simulink model "nmm2DFullBody"  (R2018a)
settings: Solver=ode23s  StartTime=0.0  StopTime=13  FixedStep=1e-3  MaxStep=ts_max  RelTol=1e-3  AbsTol=1e-4  EnableMultiTasking=on
InitFcn:
  | addpath('../lib');
  | addpath('./init_script');
  | nms_model_MechInit
  | nms_model_ControlInit
StopFcn:
  | mRFX = struct;
  | 
  | mRFX.RStance = DataFromModel.Data(:,2)
  | mRFX.RGRF_AP = DataFromModel.Data(:,24)
  | mRFX.RGRF_VT = DataFromModel.Data(:,22)
  | mRFX.RAnkleAngle = DataFromModel.Data(:,8)
  | mRFX.RKneeAngle = DataFromModel.Data(:,7)
  | mRFX.RHipAngle = DataFromModel.Data(:,6)
  | mRFX.RAnkleTorque = DataFromModel.Data(:,20)
  | mRFX.RKneeTorque = DataFromModel.Data(:,19)
  | mRFX.RHipTorque = DataFromModel.Data(:,18)
  | 
  | mRFX.RMuscleGLU = DataFromModel.Data(:,32)
  | mRFX.RMuscleHF = DataFromModel.Data(:,33)
  | mRFX.RMuscleHAM = DataFromModel.Data(:,34)
  | mRFX.RMuscleVAS = DataFromModel.Data(:,35)
  | mRFX.RMuscleGAS = DataFromModel.Data(:,36)
  | mRFX.RMuscleSOL = DataFromModel.Data(:,37)
  | mRFX.RMuscleTA = DataFromModel.Data(:,38)
  | 
  | mRFX.LStance = DataFromModel.Data(:,1)
  | mRFX.LGRF_AP = DataFromModel.Data(:,23)
  | mRFX.LGRF_VT = DataFromModel.Data(:,21)
  | mRFX.LAnkleAngle = DataFromModel.Data(:,5)
  | mRFX.LKneeAngle = DataFromModel.Data(:,4)
  | mRFX.LHipAngle = DataFromModel.Data(:,3)
  | mRFX.LAnkleTorque = DataFromModel.Data(:,17)
  | mRFX.LKneeTorque = DataFromModel.Data(:,16)
  | mRFX.LHipTorque = DataFromModel.Data(:,15)
  | 
  | mRFX.LMuscleGLU = DataFromModel.Data(:,25)
  | mRFX.LMuscleHF = DataFromModel.Data(:,26)
  | mRFX.LMuscleHAM = DataFromModel.Data(:,27)
  | mRFX.LMuscleVAS = DataFromModel.Data(:,28)
  | mRFX.LMuscleGAS = DataFromModel.Data(:,29)
  | mRFX.LMuscleSOL = DataFromModel.Data(:,30)
  | mRFX.LMuscleTA = DataFromModel.Data(:,31)
undefined symbols (not defined in the file or in its folder): alphaFmGas, alphaFmGlu, alphaFmHam, alphaFmSol, alphaFmVas, alphaLceHam, alphaLceHfl, alphaLceTa, alphaLceTa1, Amp, amp_var, c, c_jointstop, D12_F, D12_S, D12_T, D13_F, D1G_F, D1G_HAT, D1G_S, D1G_T, DeltaThRef, eref, FmaxGAS, FmaxGLU, FmaxHAM, FmaxHFL, FmaxSOL, FmaxTA, FmaxVAS, freq, freq_var, GainDeltaTheta, GainGAS, GainGLU, GainHAM, GainHAMHFL, GainHFL, GainKneOverExt, GainSOL, GainSOLTA, GainTA, GainVAS, In_F, In_HAT, In_S, In_T, K, k_gx, k_gy, k_pressure, K_swing, LceOffsetHAM, LceOffsetHFL, LceOffsetTA, LongDelay, loptGAS, loptGLU, loptHAM, loptHFL ... (+83)
libraries: nmc x77, mblibv1 x60, simulink x33, simulink_extras x18
(part 1 of 8)
settings Model: SimulationMode=accelerator  Creator=hgeyer  LastModifiedBy=Alice
settings SolverCC: AutoScaleAbsTol=off
settings DataIOCC: LimitDataPoints=on  MaxDataPoints=2500  SaveFormat=Array  SignalLoggingSaveFormat=ModelDataLogs  SaveState=on  SignalLogging=off  StateSaveName=xoutNew  OutputSaveName=youtNew
settings OptimizationCC: BooleanDataType=off  ExpressionDepthLimit=2147483647  InitFltsAndDblsToZero=on  EfficientMapNaN2IntZero=off  LifeSpan=inf
settings DebuggingCC: SaveWithParameterizedLinksMsg=none  UnderspecifiedInitializationDetection=Classic  MergeDetectMultiDrivingBlocksExec=none  SignalResolutionControl=TryResolveAllWithWarning  SolverPrmCheckMsg=warning  MultiTaskDSMMsg=warning  MultiTaskCondExecSysMsg=none  FcnCallInpInsideContextMsg=warning  AllowSymbolicDim=off  StateNameClashWarn=warning  SFUnexpectedBacktrackingDiag=warning  SFNoUnconditionalDefaultTransitionDiag=warning  SFExecutionAtInitializationDiag=none
settings HardwareCC: ProdBitPerPointer=32  ProdBitPerSizeT=32  ProdBitPerPtrDiffT=32  ProdLargestAtomicFloat=None  ProdIntDivRoundTo=Undefined  ProdEndianess=Unspecified  ProdWordSize=32  ProdHWDeviceType=32-bit Generic  TargetBitPerPointer=64  TargetBitPerSizeT=64  TargetBitPerPtrDiffT=64  TargetLongLongMode=on  TargetIntDivRoundTo=Zero  TargetEndianess=LittleEndian  TargetWordSize=64  TargetHWDeviceType=MATLAB Host  ProdEqTarget=off
settings ModelReferenceCC: PropagateSignalLabelsOutOfModel=off
settings CodeAppCC: MaxIdLength=128  StateflowObjectComments=on
settings GRTTargetCC: TargetLangStandard=C89/C90 (ANSI)  CombineOutputUpdateFcns=off  GRTInterface=on
settings ConfigComp: CovMetricSettings=dw  CovHtmlReporting=on  CovSaveCumulativeToWorkspaceVar=on  CovSaveSingleToWorkspaceVar=on  CovExternalEMLEnable=off  CovSFcnEnable=off
settings SimMechanicsCC: VisDuringSimulation=on  VisSampleTime=0.01  AutoFitVis=TIGHTFIT  LastVizWinPosition=[551 264 570 413]  CamPosition=[16.8615;0.833613;11.9413;]  CamTarget=[16.8615;0.833613;0;]  CamUpVector=[0;1;0;]  CamHeight=1.70989  VisBackgroundColor=[0.9;0.9;0.95;]  DefaultBodyColor=[1;0;0;]
settings ConfigurationSet: Description=SimMechanics 2G

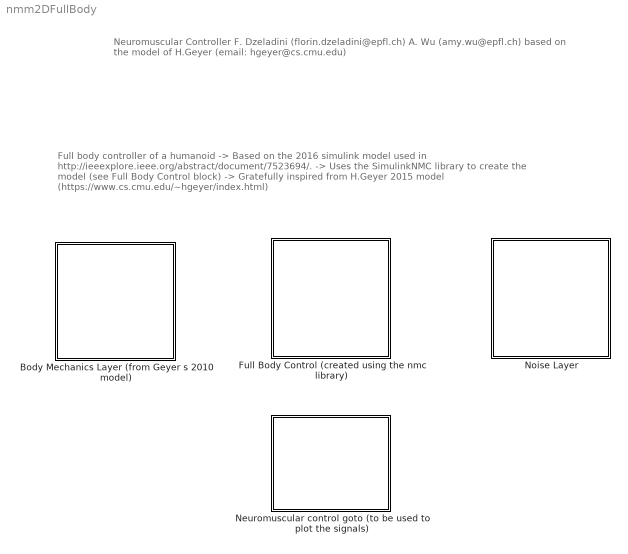
== system nmm2DFullBody ==
  note: Full body controller of a humanoid
      | -> Based on the 2016 simulink model used  in http://ieeexplore.ieee.org/abstract/document/7523694/.
      | -> Uses the SimulinkNMC library to create the model (see Full Body Control block)
      | -> Gratefully inspired from H.Geyer 2015 model (https://www.cs.cmu.edu/~hgeyer/index.html)
  note: Neuromuscular Controller
      | F. Dzeladini (florin.dzeladini@epfl.ch)
      | A. Wu (amy.wu@epfl.ch)
      | based on the model of H.Geyer (email: hgeyer@cs.cmu.edu)
  Body Mechanics Layer (from Geyer s 2010 model) : Subsystem
  Full Body Control (created using the nmc library) : Subsystem
  Neuromuscular control goto (to be used to plot the signals) : Subsystem
  Noise Layer : Subsystem

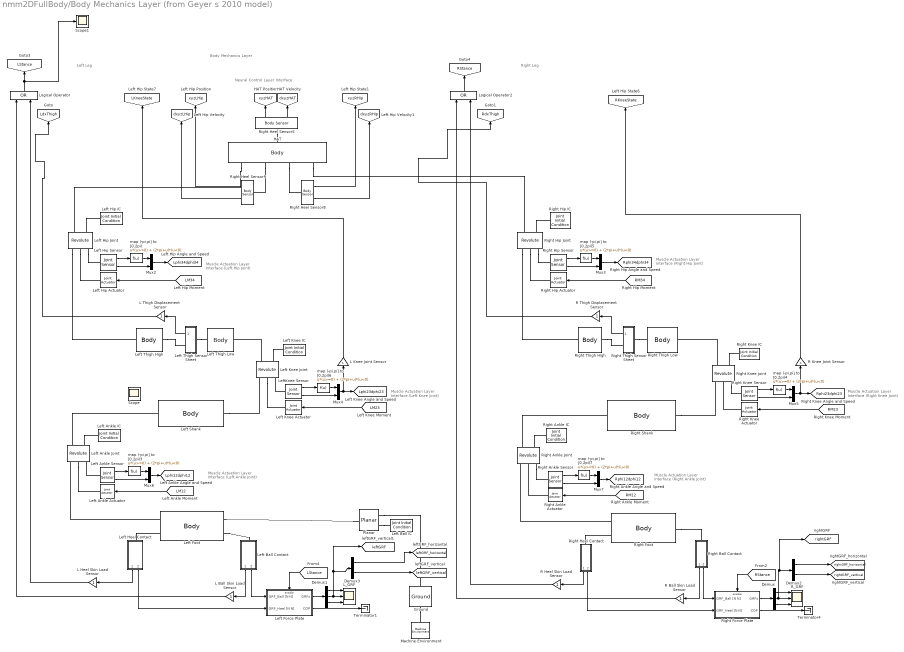
== system nmm2DFullBody/Body Mechanics Layer (from Geyer s 2010 model) ==
  note: Body Mechanics Layer
  note: Left Leg
  note: Right Leg
  note: Muscle Actuation
      | Layer Interface
      | (Left Hip Joint)
  note: Muscle Actuation
      | Layer Interface
      | (Right Hip Joint)
  note: Muscle Actuation
      | Layer Interface
      | (Right Knee Joint)
  note: Muscle Actuation
      | Layer Interface
      | (Left Knee Joint)
  note: Muscle Actuation
      | Layer Interface
      | (Left Ankle Joint)
  note: Muscle Actuation
      | Layer Interface
      | (Right Ankle Joint)
  note: Neural Control Layer Interface
  Demux : Demux  Outputs=3
  Demux1 : Demux  Outputs=3
  Demux2 : Demux  Outputs=2
  Demux3 : Demux  Outputs=2
  Ground : mblibv1/Bodies/Ground  UpdateFromCAD=off  LeftPortType=env  RightPortType=workingframe  PhysicalDomain=Mechanical  DialogClass=GroundBlock  CoordPosition=[0 0 0]  CoordPositionUnits=m  StateVectorMgrId=0  MachineId=[1 0]  ShowEnvPort=on  ParameterChecksum=[2736536609, 93968053, 2479305892, 4269051790]  TopologyChecksum=[3491173193, 3815139956, 2150979500, 405105691]
      settings: SourceProductName=Simscape  SourceProductBaseCode=SS
  HAT : mblibv1/Bodies/Body  LConnTagsString=CG  RConnTagsString=CS1|CS2|CS3|CS4  UpdateFromCAD=off  DialogClass=MechanicalBodyBlock  Mass=m_HAT  MassUnits=kg  InertiaUnits=kg*m^2  Inertia=In_HAT*[0 0 0; 0 0 0; 0 0 1]  Shape=Cylinder  ShapeDims=[1 1]  ShapeUnits=m  ShapeUse=false  Density=1  DensityUnits=kg/m^3  DensityUse=false  GraphicsMode=MACHINE_DEFAULT  BodyColorSelMode=MACHINE_DEFAULT  BodyColor=[1 0 0]  AttachedToCS=CG  CG=Left$CG$[D1G_HAT 0 0]$CS1$CS1$m$[0 0 0]$Euler X-Y-Z$deg$WORLD$true$none  WorkingFrames=Right$CS1$[0 0 0]$ADJOINING$ADJOINING$m$[0 0 0]$Euler X-Y-Z$deg$WORLD$true$none#Right$CS2$[0 0 0]$CS1$CS1$m$[0 0 0]$Euler X-Y-Z$deg$WORLD$true$none#Right$CS3$[0 0 0]$CS1$CS1$m$[0 0 0]$Euler X-Y-Z$deg$WORLD$true$none#Right$CS4$[0 0 0]$CS1$CS1$m$[0 0 0]$Euler X-Y-Z$deg$WORLD$true$none#Left$CS5$[2*D1G_HAT 0 0]$CS1$CS1$m$[0 0 0]$Euler X-Y-Z$deg$WORLD$false$none  CGPos=[D1G_HAT 0 0]  CGRot=[0 0 0]  CS0Pos=[]  CS0Rot=[]  CS1Pos=[0 0 0]  CS1Rot=[0 0 0]  CS2Pos=[0 0 0]  CS2Rot=[0 0 0]  CS3Pos=[0 0 0]  CS3Rot=[0 0 0]  CS4Pos=[0 0 0]  CS4Rot=[0 0 0]  CS5Pos=[2*D1G_HAT 0 0]  CS5Rot=[0 0 0]  CS6Pos=[]  CS6Rot=[]  CS7Pos=[]  CS7Rot=[]  CS8Pos=[]  CS8Rot=[]  CS9Pos=[]  CS9Rot=[]  CS10Pos=[]  CS10Rot=[]  CS11Pos=[]  CS11Rot=[]  CS12Pos=[]  CS12Rot=[]  CS13Pos=[]  CS13Rot=[]  CS14Pos=[]  CS14Rot=[]  CS15Pos=[]  CS15Rot=[]  CS16Pos=[]  CS16Rot=[]  CS17Pos=[]  CS17Rot=[]  CS18Pos=[]  CS18Rot=[]  CS19Pos=[]  CS19Rot=[]  CS20Pos=[]  CS20Rot=[]
      settings: SourceProductName=Simscape  SourceProductBaseCode=SS
  L Ball Skin Load Sensor : Gain
  L Heel Skin Load Sensor : Gain
  L Knee Joint Sensor : Gain
  L Thigh Displacement  Sensor : Gain
  L_GRF : Scope  NumInputPorts=3
  Left Ankle Joint : mblibv1/Joints/Revolute  LConnTagsString=__newl0|SA1|SA2  RConnTagsString=__newr0|SA1  UpdateFromCAD=off  NumSAPorts=3  CutJoint=off  MarkAsCut=off  Primitives=revolute  PrimitiveProps=R1$WORLD$[0 0 1]$revolute  DialogClass=JointBlock  R1Axis=[0 0 1]
      settings: SourceProductName=Simscape  SourceProductBaseCode=SS
  Left Ball Contact : Subsystem
  Left Heel Contact : Subsystem
  Left Hip Joint : mblibv1/Joints/Revolute  LConnTagsString=__newl0|SA1|SA2  RConnTagsString=__newr0|SA1  UpdateFromCAD=off  NumSAPorts=3  CutJoint=off  MarkAsCut=off  Primitives=revolute  PrimitiveProps=R1$WORLD$[0 0 1]$revolute  DialogClass=JointBlock  R1Axis=[0 0 1]
      settings: SourceProductName=Simscape  SourceProductBaseCode=SS
  Left Knee Joint : mblibv1/Joints/Revolute  LConnTagsString=__newl0|SA1|SA2  RConnTagsString=__newr0|SA1  UpdateFromCAD=off  NumSAPorts=3  CutJoint=off  MarkAsCut=off  Primitives=revolute  PrimitiveProps=R1$WORLD$[0 0 -1]$revolute  DialogClass=JointBlock  R1Axis=[0 0 -1]
      settings: SourceProductName=Simscape  SourceProductBaseCode=SS
  Left Ankle Actuator : mblibv1/Sensors &  Actuators/Joint Actuator  UpdateFromCAD=off  PhysicalDomain=Mechanical  PortType=blob  ActuationStyle=Force  AngleUnits=deg  ArcVelocityUnits=deg/s  ArcAccelerationUnits=deg/s^2  CoordPositionUnits=m  VelocityUnits=m/s  AccelerationUnits=m/s^2  ForceUnits=N  TorqueUnits=N-m  ActiveIO=on  Width=1  DialogClass=MechanicalActuatorBlock  Primitive=R1  ReferenceFrame=Absolute (INERTIAL)
      settings: SourceProductName=Simscape  SourceProductBaseCode=SS
  Left Ankle Sensor : mblibv1/Sensors &  Actuators/Joint Sensor  UpdateFromCAD=off  PhysicalDomain=Mechanical  PortType=blob  Muxed=off  Pose=off  Angle=on  AngleUnits=rad  ArcVelocity=on  ArcVelocityUnits=rad/s  ArcAcceleration=off  ArcAccelerationUnits=deg/s^2  CoordPosition=on  CoordPositionUnits=m  Velocity=off  VelocityUnits=m/s  Acceleration=off  AccelerationUnits=m/s^2  Quaternion=on  QuaternionDT=off  QuaternionDDT=off  QuaternionUnits=off  OutputVector=[ 1 1 ]  ActiveIO=on  Width=2  DialogClass=MechanicalSensorBlock  Primitive=R1  Force=off  ForceUnits=N  Torque=off  TorqueUnits=N-m  ReferenceFrame=Absolute (INERTIAL)  ReactionSensedSide=Base  ReactionReferenceFrame=Absolute (World)  ReactionForce=off  ReactionForceUnits=N  ReactionMoment=off  ReactionMomentUnits=N-m
      settings: SourceProductName=Simscape  SourceProductBaseCode=SS
  Left Ankle IC : mblibv1/Sensors &  Actuators/Joint Initial Condition  UpdateFromCAD=off  LeftPortType=blob  RightPortType=blob  PhysicalDomain=mechanical  DialogClass=InitialConditionBlock  InitialConditions=P1$false$0$m$rad$0$m/s$rad/s#P2$false$0$m$rad$0$m/s$rad/s#P3$false$0$m$rad$0$m/s$rad/s#R1$true$Lphi120$m$rad$0$m/s$rad/s#R2$false$0$m$rad$0$m/s$rad/s#R3$false$0$m$rad$0$m/s$rad/s#S$false$0$m$rad$0$m/s$rad/s  P1PIC=0  P1VIC=0  P2PIC=0  P2VIC=0  P3PIC=0  P3VIC=0  R1PIC=Lphi120  R1VIC=0  R2PIC=0  R2VIC=0  R3PIC=0  R3VIC=0  SPIC=0  SVIC=0
      settings: SourceProductName=Simscape  SourceProductBaseCode=SS
  Left Ball IC : mblibv1/Sensors &  Actuators/Joint Initial Condition  UpdateFromCAD=off  LeftPortType=blob  RightPortType=blob  PhysicalDomain=Mechanical  DialogClass=InitialConditionBlock  InitialConditions=P1$true$0$m$rad$vx0$m/s$rad/s#P2$true$0$m$rad$0$m/s$rad/s#P3$false$0$m$rad$0$m/s$rad/s#R1$false$0$m$rad$0$m/s$rad/s#R2$false$0$m$rad$0$m/s$rad/s#R3$false$0$m$rad$0$m/s$rad/s#S$false$0$m$rad$0$m/s$rad/s  P1PIC=0  P1VIC=vx0  P2PIC=0  P2VIC=0  P3PIC=0  P3VIC=0  R1PIC=0  R1VIC=0  R2PIC=0  R2VIC=0  R3PIC=0  R3VIC=0  SPIC=0  SVIC=0
      settings: SourceProductName=Simscape  SourceProductBaseCode=SS
  Left Foot : mblibv1/Bodies/Body  LConnTagsString=CS1|CS4  RConnTagsString=CS2|CS3  UpdateFromCAD=off  DialogClass=MechanicalBodyBlock  Mass=m_F  MassUnits=kg  InertiaUnits=kg*m^2  Inertia=[0 0 0; 0 0 0; 0 0 In_F]  Shape=Cylinder  ShapeDims=[1 1]  ShapeUnits=m  ShapeUse=false  Density=1  DensityUnits=kg/m^3  DensityUse=false  GraphicsMode=MACHINE_DEFAULT  BodyColorSelMode=MACHINE_DEFAULT  BodyColor=[1 0 0]  AttachedToCS=CG  CG=Left$CG$[-D1G_F 0 0]$CS1$CS1$m$[0 0 0]$Euler X-Y-Z$deg$WORLD$false$none  WorkingFrames=Left$CS1$[0 0 0]$ADJOINING$ADJOINING$m$[0 0 0]$Euler X-Y-Z$deg$WORLD$true$none#Right$CS2$[-D12_F 0 0]$CS1$CS1$m$[0 0 0]$Euler X-Y-Z$deg$WORLD$true$none#Right$CS3$[-D13_F 0 0]$CS1$CS1$m$[0 0 0]$Euler X-Y-Z$deg$WORLD$true$none#Left$CS4$[0 0 0]$CS1$CS1$m$[0 0 0]$Euler X-Y-Z$deg$WORLD$true$none  CGPos=[-D1G_F 0 0]  CGRot=[0 0 0]  CS0Pos=[]  CS0Rot=[]  CS1Pos=[0 0 0]  CS1Rot=[0 0 0]  CS2Pos=[-D12_F 0 0]  CS2Rot=[0 0 0]  CS3Pos=[-D13_F 0 0]  CS3Rot=[0 0 0]  CS4Pos=[0 0 0]  CS4Rot=[0 0 0]  CS5Pos=[]  CS5Rot=[]  CS6Pos=[]  CS6Rot=[]  CS7Pos=[]  CS7Rot=[]  CS8Pos=[]  CS8Rot=[]  CS9Pos=[]  CS9Rot=[]  CS10Pos=[]  CS10Rot=[]  CS11Pos=[]  CS11Rot=[]  CS12Pos=[]  CS12Rot=[]  CS13Pos=[]  CS13Rot=[]  CS14Pos=[]  CS14Rot=[]  CS15Pos=[]  CS15Rot=[]  CS16Pos=[]  CS16Rot=[]  CS17Pos=[]  CS17Rot=[]  CS18Pos=[]  CS18Rot=[]  CS19Pos=[]  CS19Rot=[]  CS20Pos=[]  CS20Rot=[]
      settings: SourceProductName=Simscape  SourceProductBaseCode=SS
  Left Force Plate : Subsystem  TreatAsAtomicUnit=on
  Left Hip Actuator : mblibv1/Sensors &  Actuators/Joint Actuator  UpdateFromCAD=off  PhysicalDomain=Mechanical  PortType=blob  ActuationStyle=Force  AngleUnits=deg  ArcVelocityUnits=deg/s  ArcAccelerationUnits=deg/s^2  CoordPositionUnits=m  VelocityUnits=m/s  AccelerationUnits=m/s^2  ForceUnits=N  TorqueUnits=N-m  ActiveIO=on  Width=1  DialogClass=MechanicalActuatorBlock  Primitive=R1  ReferenceFrame=Absolute (INERTIAL)
      settings: SourceProductName=Simscape  SourceProductBaseCode=SS
  Left Hip Sensor : mblibv1/Sensors &  Actuators/Joint Sensor  UpdateFromCAD=off  PhysicalDomain=Mechanical  PortType=blob  Muxed=off  Pose=off  Angle=on  AngleUnits=rad  ArcVelocity=on  ArcVelocityUnits=rad/s  ArcAcceleration=off  ArcAccelerationUnits=deg/s^2  CoordPosition=on  CoordPositionUnits=m  Velocity=on  VelocityUnits=m/s  Acceleration=off  AccelerationUnits=m/s^2  Quaternion=on  QuaternionDT=off  QuaternionDDT=off  QuaternionUnits=off  OutputVector=[ 1 1 ]  ActiveIO=on  Width=2  DialogClass=MechanicalSensorBlock  Primitive=R1  Force=off  ForceUnits=N  Torque=off  TorqueUnits=N-m  ReferenceFrame=Absolute (INERTIAL)  ReactionSensedSide=Base  ReactionReferenceFrame=Absolute (World)  ReactionForce=off  ReactionForceUnits=N  ReactionMoment=off  ReactionMomentUnits=N-m
      settings: SourceProductName=Simscape  SourceProductBaseCode=SS
  Left Hip IC : mblibv1/Sensors &  Actuators/Joint Initial Condition  UpdateFromCAD=off  LeftPortType=blob  RightPortType=blob  PhysicalDomain=mechanical  DialogClass=InitialConditionBlock  InitialConditions=P1$false$0$m$rad$0$m/s$rad/s#P2$false$0$m$rad$0$m/s$rad/s#P3$false$0$m$rad$0$m/s$rad/s#R1$true$Lphi340$m$rad$0$m/s$rad/s#R2$false$0$m$rad$0$m/s$rad/s#R3$false$0$m$rad$0$m/s$rad/s#S$false$0$m$rad$0$m/s$rad/s  P1PIC=0  P1VIC=0  P2PIC=0  P2VIC=0  P3PIC=0  P3VIC=0  R1PIC=Lphi340  R1VIC=0  R2PIC=0  R2VIC=0  R3PIC=0  R3VIC=0  SPIC=0  SVIC=0
      settings: SourceProductName=Simscape  SourceProductBaseCode=SS
  Left Knee Actuator : mblibv1/Sensors &  Actuators/Joint Actuator  UpdateFromCAD=off  PhysicalDomain=Mechanical  PortType=blob  ActuationStyle=Force  AngleUnits=deg  ArcVelocityUnits=deg/s  ArcAccelerationUnits=deg/s^2  CoordPositionUnits=m  VelocityUnits=m/s  AccelerationUnits=m/s^2  ForceUnits=N  TorqueUnits=N-m  ActiveIO=on  Width=1  DialogClass=MechanicalActuatorBlock  Primitive=R1  ReferenceFrame=Absolute (INERTIAL)
      settings: SourceProductName=Simscape  SourceProductBaseCode=SS
  Left Knee IC : mblibv1/Sensors &  Actuators/Joint Initial Condition  UpdateFromCAD=off  LeftPortType=blob  RightPortType=blob  PhysicalDomain=mechanical  DialogClass=InitialConditionBlock  InitialConditions=P1$false$0$m$rad$0$m/s$rad/s#P2$false$0$m$rad$0$m/s$rad/s#P3$false$0$m$rad$0$m/s$rad/s#R1$true$Lphi230$m$rad$0$m/s$deg/s#R2$false$0$m$rad$0$m/s$rad/s#R3$false$0$m$rad$0$m/s$rad/s#S$false$0$m$rad$0$m/s$rad/s  P1PIC=0  P1VIC=0  P2PIC=0  P2VIC=0  P3PIC=0  P3VIC=0  R1PIC=Lphi230  R1VIC=0  R2PIC=0  R2VIC=0  R3PIC=0  R3VIC=0  SPIC=0  SVIC=0
      settings: SourceProductName=Simscape  SourceProductBaseCode=SS
  Left Shank : mblibv1/Bodies/Body  LConnTagsString=CS1  RConnTagsString=CS2  UpdateFromCAD=off  DialogClass=MechanicalBodyBlock  Mass=m_S  MassUnits=kg  InertiaUnits=kg*m^2  Inertia=[0 0 0; 0 0 0; 0 0 In_S]  Shape=Cylinder  ShapeDims=[1 1]  ShapeUnits=m  ShapeUse=false  Density=1  DensityUnits=kg/m^3  DensityUse=false  GraphicsMode=MACHINE_DEFAULT  BodyColorSelMode=MACHINE_DEFAULT  BodyColor=[1 0 0]  AttachedToCS=CG  CG=Left$CG$[D1G_S 0 0]$CS1$CS1$m$[0 0 0]$Euler X-Y-Z$deg$WORLD$false$none  WorkingFrames=Left$CS1$[0 0 0]$ADJOINING$ADJOINING$m$[0 0 0]$Euler X-Y-Z$deg$WORLD$true$none#Right$CS2$[D12_S 0 0]$CS1$CS1$m$[0 0 0]$Euler X-Y-Z$deg$WORLD$true$none  CGPos=[D1G_S 0 0]  CGRot=[0 0 0]  CS0Pos=[]  CS0Rot=[]  CS1Pos=[0 0 0]  CS1Rot=[0 0 0]  CS2Pos=[D12_S 0 0]  CS2Rot=[0 0 0]  CS3Pos=[]  CS3Rot=[]  CS4Pos=[]  CS4Rot=[]  CS5Pos=[]  CS5Rot=[]  CS6Pos=[]  CS6Rot=[]  CS7Pos=[]  CS7Rot=[]  CS8Pos=[]  CS8Rot=[]  CS9Pos=[]  CS9Rot=[]  CS10Pos=[]  CS10Rot=[]  CS11Pos=[]  CS11Rot=[]  CS12Pos=[]  CS12Rot=[]  CS13Pos=[]  CS13Rot=[]  CS14Pos=[]  CS14Rot=[]  CS15Pos=[]  CS15Rot=[]  CS16Pos=[]  CS16Rot=[]  CS17Pos=[]  CS17Rot=[]  CS18Pos=[]  CS18Rot=[]  CS19Pos=[]  CS19Rot=[]  CS20Pos=[]  CS20Rot=[]
      settings: SourceProductName=Simscape  SourceProductBaseCode=SS
  Left Thigh Sensor Sheet : Subsystem
  Left Thigh High : mblibv1/Bodies/Body  LConnTagsString=CS2  RConnTagsString=CS1  UpdateFromCAD=off  DialogClass=MechanicalBodyBlock  Mass=m_T*(1-ThPos)  MassUnits=kg  InertiaUnits=kg*m^2  Inertia=[0 0 0; 0 0 0; 0 0 In_T*(1-ThPos)^3]  Shape=Cylinder  ShapeDims=[1 1]  ShapeUnits=m  ShapeUse=false  Density=1  DensityUnits=kg/m^3  DensityUse=false  GraphicsMode=MACHINE_DEFAULT  BodyColorSelMode=MACHINE_DEFAULT  BodyColor=[1;0;0]  AttachedToCS=CG  CG=Left$CG$[-D1G_T*(1-ThPos) 0 0]$CS1$CS1$m$[0 0 0]$Euler X-Y-Z$deg$WORLD$false  WorkingFrames=Right$CS1$[0 0 0]$ADJOINING$ADJOINING$m$[0 0 0]$Euler X-Y-Z$deg$WORLD$true#Left$CS2$[-D12_T*(1-ThPos) 0 0]$CS1$CS1$m$[0 0 0]$Euler X-Y-Z$deg$WORLD$true  CGPos=[-D1G_T*(1-ThPos) 0 0]  CGRot=[0 0 0]  CS0Pos=[]  CS0Rot=[]  CS1Pos=[0 0 0]  CS1Rot=[0 0 0]  CS2Pos=[-D12_T*(1-ThPos) 0 0]  CS2Rot=[0 0 0]  CS3Pos=[]  CS3Rot=[]  CS4Pos=[]  CS4Rot=[]  CS5Pos=[]  CS5Rot=[]  CS6Pos=[]  CS6Rot=[]  CS7Pos=[]  CS7Rot=[]  CS8Pos=[]  CS8Rot=[]  CS9Pos=[]  CS9Rot=[]  CS10Pos=[]  CS10Rot=[]  CS11Pos=[]  CS11Rot=[]  CS12Pos=[]  CS12Rot=[]  CS13Pos=[]  CS13Rot=[]  CS14Pos=[]  CS14Rot=[]  CS15Pos=[]  CS15Rot=[]  CS16Pos=[]  CS16Rot=[]  CS17Pos=[]  CS17Rot=[]  CS18Pos=[]  CS18Rot=[]  CS19Pos=[]  CS19Rot=[]  CS20Pos=[]  CS20Rot=[]
      settings: SourceProductName=Simscape  SourceProductBaseCode=SS
  Left Thigh Low : mblibv1/Bodies/Body  LConnTagsString=CS2  RConnTagsString=CS1  UpdateFromCAD=off  DialogClass=MechanicalBodyBlock  Mass=m_T*ThPos  MassUnits=kg  InertiaUnits=kg*m^2  Inertia=[0 0 0; 0 0 0; 0 0 In_T*(ThPos)^3]  Shape=Cylinder  ShapeDims=[1 1]  ShapeUnits=m  ShapeUse=false  Density=1  DensityUnits=kg/m^3  DensityUse=false  GraphicsMode=MACHINE_DEFAULT  BodyColorSelMode=MACHINE_DEFAULT  BodyColor=[1 0 0]  AttachedToCS=CG  CG=Left$CG$[-D1G_T*ThPos 0 0]$CS1$CS1$m$[0 0 0]$Euler X-Y-Z$deg$WORLD$false$none  WorkingFrames=Right$CS1$[0 0 0]$ADJOINING$ADJOINING$m$[0 0 0]$Euler X-Y-Z$deg$WORLD$true$none#Left$CS2$[-D12_T*ThPos 0 0]$CS1$CS1$m$[0 0 0]$Euler X-Y-Z$deg$WORLD$true$none  CGPos=[-D1G_T*ThPos 0 0]  CGRot=[0 0 0]  CS0Pos=[]  CS0Rot=[]  CS1Pos=[0 0 0]  CS1Rot=[0 0 0]  CS2Pos=[-D12_T*ThPos 0 0]  CS2Rot=[0 0 0]  CS3Pos=[]  CS3Rot=[]  CS4Pos=[]  CS4Rot=[]  CS5Pos=[]  CS5Rot=[]  CS6Pos=[]  CS6Rot=[]  CS7Pos=[]  CS7Rot=[]  CS8Pos=[]  CS8Rot=[]  CS9Pos=[]  CS9Rot=[]  CS10Pos=[]  CS10Rot=[]  CS11Pos=[]  CS11Rot=[]  CS12Pos=[]  CS12Rot=[]  CS13Pos=[]  CS13Rot=[]  CS14Pos=[]  CS14Rot=[]  CS15Pos=[]  CS15Rot=[]  CS16Pos=[]  CS16Rot=[]  CS17Pos=[]  CS17Rot=[]  CS18Pos=[]  CS18Rot=[]  CS19Pos=[]  CS19Rot=[]  CS20Pos=[]  CS20Rot=[]
      settings: SourceProductName=Simscape  SourceProductBaseCode=SS
  LeftKnee Sensor : mblibv1/Sensors &  Actuators/Joint Sensor  UpdateFromCAD=off  PhysicalDomain=Mechanical  PortType=blob  Muxed=off  Pose=off  Angle=on  AngleUnits=rad  ArcVelocity=on  ArcVelocityUnits=rad/s  ArcAcceleration=off  ArcAccelerationUnits=deg/s^2  CoordPosition=on  CoordPositionUnits=m  Velocity=off  VelocityUnits=m/s  Acceleration=off  AccelerationUnits=m/s^2  Quaternion=on  QuaternionDT=off  QuaternionDDT=off  QuaternionUnits=off  OutputVector=[ 1 1 ]  ActiveIO=on  Width=2  DialogClass=MechanicalSensorBlock  Primitive=R1  Force=off  ForceUnits=N  Torque=off  TorqueUnits=N-m  ReferenceFrame=Absolute (INERTIAL)  ReactionSensedSide=Base  ReactionReferenceFrame=Absolute (World)  ReactionForce=off  ReactionForceUnits=N  ReactionMoment=off  ReactionMomentUnits=N-m
      settings: SourceProductName=Simscape  SourceProductBaseCode=SS
  Logical Operator : Logic  Operator=OR  AllPortsSameDT=off  OutDataTypeStr=boolean
  Logical Operator2 : Logic  Operator=OR  AllPortsSameDT=off  OutDataTypeStr=boolean
  Machine Environment : mblibv1/Bodies/Machine Environment  Tag=Factory ground  PortType=env  PhysicalDomain=Mechanical  DialogTemplateClass=MECH.MachineEnvironment  SyncWhenCopied=off  Gravity=[0 -9.81 0]  GravityUnits=m/s^2  GravityAsSignal=off  Dimensionality=2D Only  AnalysisType=Forward dynamics  LinearAssemblyTolerance=1e-3  LinearAssemblyToleranceUnits=m  AngularAssemblyTolerance=1e-3  AngularAssemblyToleranceUnits=rad  ConstraintSolverType=Tolerancing  ConstraintRelTolerance=1e-3  ConstraintAbsTolerance=1e-3  UseRobustSingularityHandling=off  RedundancyAnalysisToleranceType=Automatically select tolerance  RedundancyAnalysisTolerance=1e-14  StatePerturbationType=Fixed  PerturbationSize=1e-3  VisualizeMachine=on  BodyVisualizationType=Use model default body geometries  BodyColorSelMode=Use model default  DefaultBodyColor=[1 0 0]
      settings: SourceProductName=Simscape  SourceProductBaseCode=SS
  Mux{2..7} (6 alike) : Mux  Inputs=2
  Planar : mblibv1/Joints/Planar  LConnTagsString=__newl0|SA1  RConnTagsString=__newr0  UpdateFromCAD=off  NumSAPorts=1  CutJoint=off  MarkAsCut=off  Primitives=prismatic_prismatic_revolute  PrimitiveProps=P1$WORLD$[1 0 0]$prismatic#P2$WORLD$[0 1 0]$prismatic#R1$WORLD$[0 0 1]$revolute  DialogClass=JointBlock  P1Axis=[1 0 0]  P2Axis=[0 1 0]  R1Axis=[0 0 1]
      settings: SourceProductName=Simscape  SourceProductBaseCode=SS
  R Ball Skin Load Sensor : Gain
  R Heel Skin Load Sensor : Gain
  R Knee Joint Sensor : Gain
  R Thigh Displacement  Sensor : Gain
  R_GRF : Scope  NumInputPorts=3
  Right Ankle Joint : mblibv1/Joints/Revolute  LConnTagsString=__newl0|SA1|SA2  RConnTagsString=__newr0|SA1  UpdateFromCAD=off  NumSAPorts=3  CutJoint=off  MarkAsCut=off  Primitives=revolute  PrimitiveProps=R1$WORLD$[0 0 1]$revolute  DialogClass=JointBlock  R1Axis=[0 0 1]
      settings: SourceProductName=Simscape  SourceProductBaseCode=SS
  Right Ball Contact : Subsystem
  Right Heel Contact : Subsystem
  Right Hip Joint : mblibv1/Joints/Revolute  LConnTagsString=__newl0|SA1|SA2  RConnTagsString=__newr0|SA1  UpdateFromCAD=off  NumSAPorts=3  CutJoint=off  MarkAsCut=off  Primitives=revolute  PrimitiveProps=R1$WORLD$[0 0 1]$revolute  DialogClass=JointBlock  R1Axis=[0 0 1]
      settings: SourceProductName=Simscape  SourceProductBaseCode=SS
  Right Knee Joint : mblibv1/Joints/Revolute  LConnTagsString=__newl0|SA1|SA2  RConnTagsString=__newr0|SA1  UpdateFromCAD=off  NumSAPorts=3  CutJoint=off  MarkAsCut=off  Primitives=revolute  PrimitiveProps=R1$WORLD$[0 0 -1]$revolute  DialogClass=JointBlock  R1Axis=[0 0 -1]
      settings: SourceProductName=Simscape  SourceProductBaseCode=SS
  Right Ankle Actuator : mblibv1/Sensors &  Actuators/Joint Actuator  UpdateFromCAD=off  PhysicalDomain=Mechanical  PortType=blob  ActuationStyle=Force  AngleUnits=deg  ArcVelocityUnits=deg/s  ArcAccelerationUnits=deg/s^2  CoordPositionUnits=m  VelocityUnits=m/s  AccelerationUnits=m/s^2  ForceUnits=N  TorqueUnits=N-m  ActiveIO=on  Width=1  DialogClass=MechanicalActuatorBlock  Primitive=R1  ReferenceFrame=Absolute (INERTIAL)
      settings: SourceProductName=Simscape  SourceProductBaseCode=SS
  Right Ankle Sensor : mblibv1/Sensors &  Actuators/Joint Sensor  UpdateFromCAD=off  PhysicalDomain=Mechanical  PortType=blob  Muxed=off  Pose=off  Angle=on  AngleUnits=rad  ArcVelocity=on  ArcVelocityUnits=rad/s  ArcAcceleration=off  ArcAccelerationUnits=deg/s^2  CoordPosition=on  CoordPositionUnits=m  Velocity=off  VelocityUnits=m/s  Acceleration=off  AccelerationUnits=m/s^2  Quaternion=on  QuaternionDT=off  QuaternionDDT=off  QuaternionUnits=off  OutputVector=[ 1 1 ]  ActiveIO=on  Width=2  DialogClass=MechanicalSensorBlock  Primitive=R1  Force=off  ForceUnits=N  Torque=off  TorqueUnits=N-m  ReferenceFrame=Absolute (INERTIAL)  ReactionSensedSide=Base  ReactionReferenceFrame=Absolute (World)  ReactionForce=off  ReactionForceUnits=N  ReactionMoment=off  ReactionMomentUnits=N-m
      settings: SourceProductName=Simscape  SourceProductBaseCode=SS
  Right Ankle IC : mblibv1/Sensors &  Actuators/Joint Initial Condition  UpdateFromCAD=off  LeftPortType=blob  RightPortType=blob  PhysicalDomain=mechanical  DialogClass=InitialConditionBlock  InitialConditions=P1$false$0$m$rad$0$m/s$rad/s#P2$false$0$m$rad$0$m/s$rad/s#P3$false$0$m$rad$0$m/s$rad/s#R1$true$Rphi120$m$rad$0$m/s$rad/s#R2$false$0$m$rad$0$m/s$rad/s#R3$false$0$m$rad$0$m/s$rad/s#S$false$0$m$rad$0$m/s$rad/s  P1PIC=0  P1VIC=0  P2PIC=0  P2VIC=0  P3PIC=0  P3VIC=0  R1PIC=Rphi120  R1VIC=0  R2PIC=0  R2VIC=0  R3PIC=0  R3VIC=0  SPIC=0  SVIC=0
      settings: SourceProductName=Simscape  SourceProductBaseCode=SS
  Right Foot : mblibv1/Bodies/Body  LConnTagsString=CS1  RConnTagsString=CS2|CS3  UpdateFromCAD=off  DialogClass=MechanicalBodyBlock  Mass=m_F  MassUnits=kg  InertiaUnits=kg*m^2  Inertia=[0 0 0; 0 0 0; 0 0 In_F]  Shape=Cylinder  ShapeDims=[1 1]  ShapeUnits=m  ShapeUse=false  Density=1  DensityUnits=kg/m^3  DensityUse=false  GraphicsMode=MACHINE_DEFAULT  BodyColorSelMode=MACHINE_DEFAULT  BodyColor=[1 0 0]  AttachedToCS=CG  CG=Left$CG$[-D1G_F 0 0]$CS1$CS1$m$[0 0 0]$Euler X-Y-Z$deg$WORLD$false$none  WorkingFrames=Left$CS1$[0 0 0]$ADJOINING$ADJOINING$m$[0 0 0]$Euler X-Y-Z$deg$WORLD$true$none#Right$CS2$[-D12_F 0 0]$CS1$CS1$m$[0 0 0]$Euler X-Y-Z$deg$WORLD$true$none#Right$CS3$[-D13_F 0 0]$CS1$CS1$m$[0 0 0]$Euler X-Y-Z$deg$WORLD$true$none  CGPos=[-D1G_F 0 0]  CGRot=[0 0 0]  CS0Pos=[]  CS0Rot=[]  CS1Pos=[0 0 0]  CS1Rot=[0 0 0]  CS2Pos=[-D12_F 0 0]  CS2Rot=[0 0 0]  CS3Pos=[-D13_F 0 0]  CS3Rot=[0 0 0]  CS4Pos=[]  CS4Rot=[]  CS5Pos=[]  CS5Rot=[]  CS6Pos=[]  CS6Rot=[]  CS7Pos=[]  CS7Rot=[]  CS8Pos=[]  CS8Rot=[]  CS9Pos=[]  CS9Rot=[]  CS10Pos=[]  CS10Rot=[]  CS11Pos=[]  CS11Rot=[]  CS12Pos=[]  CS12Rot=[]  CS13Pos=[]  CS13Rot=[]  CS14Pos=[]  CS14Rot=[]  CS15Pos=[]  CS15Rot=[]  CS16Pos=[]  CS16Rot=[]  CS17Pos=[]  CS17Rot=[]  CS18Pos=[]  CS18Rot=[]  CS19Pos=[]  CS19Rot=[]  CS20Pos=[]  CS20Rot=[]
      settings: SourceProductName=Simscape  SourceProductBaseCode=SS
  Right Force Plate : Subsystem  TreatAsAtomicUnit=on
  Right Heel Sensor5 : mblibv1/Sensors &  Actuators/Body Sensor  UpdateFromCAD=off  PhysicalDomain=Mechanical  PortType=blob  Muxed=off  Pose=off  Angle=on  AngleUnits=deg  ArcVelocity=off  ArcVelocityUnits=deg/s  ArcAcceleration=off  ArcAccelerationUnits=deg/s^2  CoordPosition=on  CoordPositionUnits=m  Velocity=on  VelocityUnits=m/s  Acceleration=off  AccelerationUnits=m/s^2  Quaternion=on  QuaternionDT=off  QuaternionDDT=off  QuaternionUnits=off  OutputVector=[ 3 3 ]  ActiveIO=on  Width=6  DialogClass=MechanicalSensorBlock  ReferenceFrame=Absolute (World)
      settings: SourceProductName=Simscape  SourceProductBaseCode=SS
  Right Heel Sensor8 : mblibv1/Sensors &  Actuators/Body Sensor  UpdateFromCAD=off  PhysicalDomain=Mechanical  PortType=blob  Muxed=off  Pose=off  Angle=on  AngleUnits=deg  ArcVelocity=off  ArcVelocityUnits=deg/s  ArcAcceleration=off  ArcAccelerationUnits=deg/s^2  CoordPosition=on  CoordPositionUnits=m  Velocity=on  VelocityUnits=m/s  Acceleration=off  AccelerationUnits=m/s^2  Quaternion=on  QuaternionDT=off  QuaternionDDT=off  QuaternionUnits=off  OutputVector=[ 3 3 ]  ActiveIO=on  Width=6  DialogClass=MechanicalSensorBlock  ReferenceFrame=Absolute (World)
      settings: SourceProductName=Simscape  SourceProductBaseCode=SS
  Right Heel Sensor9 : mblibv1/Sensors &  Actuators/Body Sensor  UpdateFromCAD=off  PhysicalDomain=Mechanical  PortType=blob  Muxed=off  Pose=off  Angle=on  AngleUnits=deg  ArcVelocity=off  ArcVelocityUnits=deg/s  ArcAcceleration=off  ArcAccelerationUnits=deg/s^2  CoordPosition=on  CoordPositionUnits=m  Velocity=on  VelocityUnits=m/s  Acceleration=off  AccelerationUnits=m/s^2  Quaternion=on  QuaternionDT=off  QuaternionDDT=off  QuaternionUnits=off  OutputVector=[ 3 3 ]  ActiveIO=on  Width=6  DialogClass=MechanicalSensorBlock  ReferenceFrame=Absolute (World)
      settings: SourceProductName=Simscape  SourceProductBaseCode=SS
  Right Hip Actuator : mblibv1/Sensors &  Actuators/Joint Actuator  UpdateFromCAD=off  PhysicalDomain=Mechanical  PortType=blob  ActuationStyle=Force  AngleUnits=deg  ArcVelocityUnits=deg/s  ArcAccelerationUnits=deg/s^2  CoordPositionUnits=m  VelocityUnits=m/s  AccelerationUnits=m/s^2  ForceUnits=N  TorqueUnits=N-m  ActiveIO=on  Width=1  DialogClass=MechanicalActuatorBlock  Primitive=R1  ReferenceFrame=Absolute (INERTIAL)
      settings: SourceProductName=Simscape  SourceProductBaseCode=SS
  Right Hip Sensor : mblibv1/Sensors &  Actuators/Joint Sensor  UpdateFromCAD=off  PhysicalDomain=Mechanical  PortType=blob  Muxed=off  Pose=off  Angle=on  AngleUnits=rad  ArcVelocity=on  ArcVelocityUnits=rad/s  ArcAcceleration=off  ArcAccelerationUnits=deg/s^2  CoordPosition=on  CoordPositionUnits=m  Velocity=on  VelocityUnits=m/s  Acceleration=off  AccelerationUnits=m/s^2  Quaternion=on  QuaternionDT=off  QuaternionDDT=off  QuaternionUnits=off  OutputVector=[ 1 1 ]  ActiveIO=on  Width=2  DialogClass=MechanicalSensorBlock  Primitive=R1  Force=off  ForceUnits=N  Torque=off  TorqueUnits=N-m  ReferenceFrame=Absolute (INERTIAL)  ReactionSensedSide=Base  ReactionReferenceFrame=Absolute (World)  ReactionForce=off  ReactionForceUnits=N  ReactionMoment=off  ReactionMomentUnits=N-m
      settings: SourceProductName=Simscape  SourceProductBaseCode=SS
  Right Hip IC : mblibv1/Sensors &  Actuators/Joint Initial Condition  UpdateFromCAD=off  LeftPortType=blob  RightPortType=blob  PhysicalDomain=mechanical  DialogClass=InitialConditionBlock  InitialConditions=P1$false$0$m$rad$0$m/s$rad/s#P2$false$0$m$rad$0$m/s$rad/s#P3$false$0$m$rad$0$m/s$rad/s#R1$true$Rphi340$m$rad$0$m/s$rad/s#R2$false$0$m$rad$0$m/s$rad/s#R3$false$0$m$rad$0$m/s$rad/s#S$false$0$m$rad$0$m/s$rad/s  P1PIC=0  P1VIC=0  P2PIC=0  P2VIC=0  P3PIC=0  P3VIC=0  R1PIC=Rphi340  R1VIC=0  R2PIC=0  R2VIC=0  R3PIC=0  R3VIC=0  SPIC=0  SVIC=0
      settings: SourceProductName=Simscape  SourceProductBaseCode=SS
  Right Knee Actuator : mblibv1/Sensors &  Actuators/Joint Actuator  UpdateFromCAD=off  PhysicalDomain=Mechanical  PortType=blob  ActuationStyle=Force  AngleUnits=deg  ArcVelocityUnits=deg/s  ArcAccelerationUnits=deg/s^2  CoordPositionUnits=m  VelocityUnits=m/s  AccelerationUnits=m/s^2  ForceUnits=N  TorqueUnits=N-m  ActiveIO=on  Width=1  DialogClass=MechanicalActuatorBlock  Primitive=R1  ReferenceFrame=Absolute (INERTIAL)
      settings: SourceProductName=Simscape  SourceProductBaseCode=SS
  Right Knee Sensor : mblibv1/Sensors &  Actuators/Joint Sensor  UpdateFromCAD=off  PhysicalDomain=Mechanical  PortType=blob  Muxed=off  Pose=off  Angle=on  AngleUnits=rad  ArcVelocity=on  ArcVelocityUnits=rad/s  ArcAcceleration=off  ArcAccelerationUnits=deg/s^2  CoordPosition=on  CoordPositionUnits=m  Velocity=off  VelocityUnits=m/s  Acceleration=off  AccelerationUnits=m/s^2  Quaternion=on  QuaternionDT=off  QuaternionDDT=off  QuaternionUnits=off  OutputVector=[ 1 1 ]  ActiveIO=on  Width=2  DialogClass=MechanicalSensorBlock  Primitive=R1  Force=off  ForceUnits=N  Torque=off  TorqueUnits=N-m  ReferenceFrame=Absolute (INERTIAL)  ReactionSensedSide=Base  ReactionReferenceFrame=Absolute (World)  ReactionForce=off  ReactionForceUnits=N  ReactionMoment=off  ReactionMomentUnits=N-m
      settings: SourceProductName=Simscape  SourceProductBaseCode=SS
  Right Knee IC : mblibv1/Sensors &  Actuators/Joint Initial Condition  UpdateFromCAD=off  LeftPortType=blob  RightPortType=blob  PhysicalDomain=mechanical  DialogClass=InitialConditionBlock  InitialConditions=P1$false$0$m$rad$0$m/s$rad/s#P2$false$0$m$rad$0$m/s$rad/s#P3$false$0$m$rad$0$m/s$rad/s#R1$true$Rphi230$m$rad$0$m/s$rad/s#R2$false$0$m$rad$0$m/s$rad/s#R3$false$0$m$rad$0$m/s$rad/s#S$false$0$m$rad$0$m/s$rad/s  P1PIC=0  P1VIC=0  P2PIC=0  P2VIC=0  P3PIC=0  P3VIC=0  R1PIC=Rphi230  R1VIC=0  R2PIC=0  R2VIC=0  R3PIC=0  R3VIC=0  SPIC=0  SVIC=0
      settings: SourceProductName=Simscape  SourceProductBaseCode=SS
  Right Shank : mblibv1/Bodies/Body  LConnTagsString=CS1  RConnTagsString=CS2  UpdateFromCAD=off  DialogClass=MechanicalBodyBlock  Mass=m_S  MassUnits=kg  InertiaUnits=kg*m^2  Inertia=[0 0 0; 0 0 0; 0 0 In_S]  Shape=Cylinder  ShapeDims=[1 1]  ShapeUnits=m  ShapeUse=false  Density=1  DensityUnits=kg/m^3  DensityUse=false  GraphicsMode=MACHINE_DEFAULT  BodyColorSelMode=MACHINE_DEFAULT  BodyColor=[1 0 0]  AttachedToCS=CG  CG=Left$CG$[D1G_S 0 0]$CS1$CS1$m$[0 0 0]$Euler X-Y-Z$deg$WORLD$false$none  WorkingFrames=Left$CS1$[0 0 0]$ADJOINING$ADJOINING$m$[0 0 0]$Euler X-Y-Z$deg$WORLD$true$none#Right$CS2$[D12_S 0 0]$CS1$CS1$m$[0 0 0]$Euler X-Y-Z$deg$WORLD$true$none  CGPos=[D1G_S 0 0]  CGRot=[0 0 0]  CS0Pos=[]  CS0Rot=[]  CS1Pos=[0 0 0]  CS1Rot=[0 0 0]  CS2Pos=[D12_S 0 0]  CS2Rot=[0 0 0]  CS3Pos=[]  CS3Rot=[]  CS4Pos=[]  CS4Rot=[]  CS5Pos=[]  CS5Rot=[]  CS6Pos=[]  CS6Rot=[]  CS7Pos=[]  CS7Rot=[]  CS8Pos=[]  CS8Rot=[]  CS9Pos=[]  CS9Rot=[]  CS10Pos=[]  CS10Rot=[]  CS11Pos=[]  CS11Rot=[]  CS12Pos=[]  CS12Rot=[]  CS13Pos=[]  CS13Rot=[]  CS14Pos=[]  CS14Rot=[]  CS15Pos=[]  CS15Rot=[]  CS16Pos=[]  CS16Rot=[]  CS17Pos=[]  CS17Rot=[]  CS18Pos=[]  CS18Rot=[]  CS19Pos=[]  CS19Rot=[]  CS20Pos=[]  CS20Rot=[]
      settings: SourceProductName=Simscape  SourceProductBaseCode=SS
  Right Thigh Sensor Sheet : Subsystem
  Right Thigh High : mblibv1/Bodies/Body  LConnTagsString=CS2  RConnTagsString=CS1  UpdateFromCAD=off  DialogClass=MechanicalBodyBlock  Mass=m_T*(1-ThPos)  MassUnits=kg  InertiaUnits=kg*m^2  Inertia=[0 0 0; 0 0 0; 0 0 In_T*(1-ThPos)^3]  Shape=Cylinder  ShapeDims=[1 1]  ShapeUnits=m  ShapeUse=false  Density=1  DensityUnits=kg/m^3  DensityUse=false  GraphicsMode=MACHINE_DEFAULT  BodyColorSelMode=MACHINE_DEFAULT  BodyColor=[1;0;0]  AttachedToCS=CG  CG=Left$CG$[-D1G_T*(1-ThPos) 0 0]$CS1$CS1$m$[0 0 0]$Euler X-Y-Z$deg$WORLD$false  WorkingFrames=Right$CS1$[0 0 0]$ADJOINING$ADJOINING$m$[0 0 0]$Euler X-Y-Z$deg$WORLD$true#Left$CS2$[-D12_T*(1-ThPos) 0 0]$CS1$CS1$m$[0 0 0]$Euler X-Y-Z$deg$WORLD$true  CGPos=[-D1G_T*(1-ThPos) 0 0]  CGRot=[0 0 0]  CS0Pos=[]  CS0Rot=[]  CS1Pos=[0 0 0]  CS1Rot=[0 0 0]  CS2Pos=[-D12_T*(1-ThPos) 0 0]  CS2Rot=[0 0 0]  CS3Pos=[]  CS3Rot=[]  CS4Pos=[]  CS4Rot=[]  CS5Pos=[]  CS5Rot=[]  CS6Pos=[]  CS6Rot=[]  CS7Pos=[]  CS7Rot=[]  CS8Pos=[]  CS8Rot=[]  CS9Pos=[]  CS9Rot=[]  CS10Pos=[]  CS10Rot=[]  CS11Pos=[]  CS11Rot=[]  CS12Pos=[]  CS12Rot=[]  CS13Pos=[]  CS13Rot=[]  CS14Pos=[]  CS14Rot=[]  CS15Pos=[]  CS15Rot=[]  CS16Pos=[]  CS16Rot=[]  CS17Pos=[]  CS17Rot=[]  CS18Pos=[]  CS18Rot=[]  CS19Pos=[]  CS19Rot=[]  CS20Pos=[]  CS20Rot=[]
      settings: SourceProductName=Simscape  SourceProductBaseCode=SS
  Right Thigh Low : mblibv1/Bodies/Body  LConnTagsString=CS2  RConnTagsString=CS1  UpdateFromCAD=off  DialogClass=MechanicalBodyBlock  Mass=m_T*ThPos  MassUnits=kg  InertiaUnits=kg*m^2  Inertia=[0 0 0; 0 0 0; 0 0 In_T*(ThPos)^3]  Shape=Cylinder  ShapeDims=[1 1]  ShapeUnits=m  ShapeUse=false  Density=1  DensityUnits=kg/m^3  DensityUse=false  GraphicsMode=MACHINE_DEFAULT  BodyColorSelMode=MACHINE_DEFAULT  BodyColor=[1 0 0]  AttachedToCS=CG  CG=Left$CG$[-D1G_T*ThPos 0 0]$CS1$CS1$m$[0 0 0]$Euler X-Y-Z$deg$WORLD$false$none  WorkingFrames=Right$CS1$[0 0 0]$ADJOINING$ADJOINING$m$[0 0 0]$Euler X-Y-Z$deg$WORLD$true$none#Left$CS2$[-D12_T*ThPos 0 0]$CS1$CS1$m$[0 0 0]$Euler X-Y-Z$deg$WORLD$true$none  CGPos=[-D1G_T*ThPos 0 0]  CGRot=[0 0 0]  CS0Pos=[]  CS0Rot=[]  CS1Pos=[0 0 0]  CS1Rot=[0 0 0]  CS2Pos=[-D12_T*ThPos 0 0]  CS2Rot=[0 0 0]  CS3Pos=[]  CS3Rot=[]  CS4Pos=[]  CS4Rot=[]  CS5Pos=[]  CS5Rot=[]  CS6Pos=[]  CS6Rot=[]  CS7Pos=[]  CS7Rot=[]  CS8Pos=[]  CS8Rot=[]  CS9Pos=[]  CS9Rot=[]  CS10Pos=[]  CS10Rot=[]  CS11Pos=[]  CS11Rot=[]  CS12Pos=[]  CS12Rot=[]  CS13Pos=[]  CS13Rot=[]  CS14Pos=[]  CS14Rot=[]  CS15Pos=[]  CS15Rot=[]  CS16Pos=[]  CS16Rot=[]  CS17Pos=[]  CS17Rot=[]  CS18Pos=[]  CS18Rot=[]  CS19Pos=[]  CS19Rot=[]  CS20Pos=[]  CS20Rot=[]
      settings: SourceProductName=Simscape  SourceProductBaseCode=SS
  Scope : Scope
  Scope1 : Scope
  Terminator1 : Terminator
  Terminator4 : Terminator
  map (-pi,pi] to [0,2pi){,3..7} (6 alike) : Fcn  Expr=u*(u>=0) + (2*pi+u)*(u<0)
  tag scope: LKneeState=global, LStance=global, LdxThigh=global, Lphi12dphi12=global, Lphi23dphi23=global, Lphi34dphi34=global, RKneeState=global, RStance=global, RdxThigh=global, Rphi12dphi12=global, Rphi23dphi23=global, Rphi34dphi34=global, dxyzHAT=global, dxyzLHip=global, dxyzRHip=global, leftGRF=global, leftGRF_horizontal=global, leftGRF_vertical=global, rightGRF=global, rightGRF_horizontal=global, rightGRF_vertical=global, xyzHAT=global, xyzLHip=global, xyzRHip=global
  wires:
  [RStance] -> Right Force Plate/Enable
  Right Ball Contact/2(GRF [N N]) -> Right Force Plate/1("GRF_Ball [N N] ")
  Right Heel Contact/2(GRF [N N]) -> Right Force Plate/2(GRF_Heel [N N])
  Right Force Plate/1(GRFs) -> Demux/1
  Demux/1 -> R_GRF/1
  Demux/2 -> [rightGRF], Demux2/1, R_GRF/2
  Demux/3 -> R_GRF/3
  Right Force Plate/2(COP) -> Terminator4/1
  Right Heel Sensor5/1 -> [xyzHAT]
  Right Heel Sensor5/2 -> [dxyzHAT]
  [LStance] -> Left Force Plate/Enable
  Left Ball Contact/2(GRF [N N]) -> Left Force Plate/1("GRF_Ball [N N] ")
  Left Heel Contact/2(GRF [N N]) -> Left Force Plate/2(GRF_Heel [N N])
  Left Force Plate/1(GRFs) -> Demux1/1
  Demux1/1 -> L_GRF/1
  Demux1/2 -> [leftGRF], Demux3/1, L_GRF/2
  Demux1/3 -> L_GRF/3
  Left Force Plate/2(COP) -> Terminator1/1
  [RM12] -> Right Ankle Actuator/1
  [RM23] -> Right Knee Actuator/1
  [RM34] -> Right Hip Actuator/1
  [LM12] -> Left Ankle Actuator/1
  [LM23] -> Left Knee Actuator/1
  [LM34] -> Left Hip Actuator/1
  Right Heel Sensor9/1 -> [xyzLHip]
  Right Heel Sensor9/2 -> [dxyzLHip]
  Right Heel Sensor8/2 -> [dxyzRHip]
  Right Heel Sensor8/1 -> [xyzRHip]
  Left Heel Contact/1(LHeelCnt) -> L Heel Skin Load Sensor/1
  L Heel Skin Load Sensor/1 -> Logical Operator/2
  L Ball Skin Load Sensor/1 -> Logical Operator/1
  Left Ball Contact/1(LBallCnt) -> L Ball Skin Load Sensor/1
  R Heel Skin Load Sensor/1 -> Logical Operator2/2
  Right Heel Contact/1(RHeelCnt) -> R Heel Skin Load Sensor/1
  Right Ball Contact/1(RBallCnt) -> R Ball Skin Load Sensor/1
  R Ball Skin Load Sensor/1 -> Logical Operator2/1
  Left Thigh Sensor Sheet/1(dx) -> L Thigh Displacement  Sensor/1
  L Thigh Displacement  Sensor/1 -> [LdxThigh]
  Right Thigh Sensor Sheet/1(dx) -> R Thigh Displacement  Sensor/1
  R Thigh Displacement  Sensor/1 -> [RdxThigh]
  map (-pi,pi] to [0,2pi)/1 -> Mux2/1
  Left Hip Sensor/2 -> Mux2/2
  Left Hip Sensor/1 -> map (-pi,pi] to [0,2pi)/1
  Mux2/1 -> [Lphi34dphi34]
  map (-pi,pi] to [0,2pi)5/1 -> Mux3/1
  Right Hip Sensor/2 -> Mux3/2
  Right Hip Sensor/1 -> map (-pi,pi] to [0,2pi)5/1
  Mux3/1 -> [Rphi34dphi34]
  map (-pi,pi] to [0,2pi)6/1 -> Mux4/1
  LeftKnee Sensor/2 -> Mux4/2
  LeftKnee Sensor/1 -> map (-pi,pi] to [0,2pi)6/1
  Mux4/1 -> [Lphi23dphi23], L Knee Joint Sensor/1
  map (-pi,pi] to [0,2pi)4/1 -> Mux5/1
  Right Knee Sensor/2 -> Mux5/2
  Mux5/1 -> [Rphi23dphi23], R Knee Joint Sensor/1
  Right Knee Sensor/1 -> map (-pi,pi] to [0,2pi)4/1
  map (-pi,pi] to [0,2pi)3/1 -> Mux6/1
  Left Ankle Sensor/2 -> Mux6/2
  Left Ankle Sensor/1 -> map (-pi,pi] to [0,2pi)3/1
  Mux6/1 -> [Lphi12dphi12]
  map (-pi,pi] to [0,2pi)7/1 -> Mux7/1
  Right Ankle Sensor/2 -> Mux7/2
  Right Ankle Sensor/1 -> map (-pi,pi] to [0,2pi)7/1
  Mux7/1 -> [Rphi12dphi12]
  L Knee Joint Sensor/1 -> [LKneeState]
  R Knee Joint Sensor/1 -> [RKneeState]
  Demux2/2 -> [rightGRF_vertical]
  Demux3/2 -> [leftGRF_vertical]
  Demux2/1 -> [rightGRF_horizontal]
  Logical Operator/1 -> Scope1/1, [LStance]
  Logical Operator2/1 -> [RStance]
  Demux3/1 -> [leftGRF_horizontal]
  connections:
  HAT/RConn1 -- Left Hip Joint/RConn1
  Left Foot/RConn1 -- Left Ankle Joint/LConn1
  Left Ankle Joint/LConn2 -- Left Ankle Actuator/RConn1
  Left Ankle Sensor/LConn1 -- Left Ankle Joint/LConn3
  Left Ankle Joint/RConn1 -- Left Shank/LConn1
  Left Ankle Joint/RConn2 -- Left Ankle IC/RConn1
  Left Heel Contact/LConn1 -- Left Foot/RConn2
  Left Hip Joint/LConn1 -- Left Thigh High/LConn1
  Left Hip Joint/LConn2 -- Left Hip Actuator/RConn1
  Left Hip Joint/LConn3 -- Left Hip Sensor/LConn1
  Left Hip Joint/RConn2 -- Left Hip IC/RConn1
  Left Shank/RConn1 -- Left Knee Joint/LConn1
  Left Knee Joint/LConn2 -- Left Knee Actuator/RConn1
  LeftKnee Sensor/LConn1 -- Left Knee Joint/LConn3
  Left Knee Joint/RConn1 -- Left Thigh Low/RConn1
  Left Knee Joint/RConn2 -- Left Knee IC/RConn1
  Left Thigh Sensor Sheet/LConn1 -- Left Thigh Low/LConn1
  Left Thigh High/RConn1 -- Left Thigh Sensor Sheet/RConn1
  Right Foot/RConn1 -- Right Ankle Joint/LConn1
  Right Ankle Actuator/RConn1 -- Right Ankle Joint/LConn2
  Right Ankle Joint/LConn3 -- Right Ankle Sensor/LConn1
  Right Ankle Joint/RConn1 -- Right Shank/LConn1
  Right Ankle Joint/RConn2 -- Right Ankle IC/RConn1
  Right Foot/LConn1 -- Right Ball Contact/LConn1
  Right Heel Contact/LConn1 -- Right Foot/RConn2
  Right Hip Joint/LConn1 -- Right Thigh High/LConn1
  Right Hip Joint/LConn2 -- Right Hip Actuator/RConn1
  Right Hip Joint/LConn3 -- Right Hip Sensor/LConn1
  Right Hip IC/RConn1 -- Right Hip Joint/RConn2
  Right Shank/RConn1 -- Right Knee Joint/LConn1
  Right Knee Actuator/RConn1 -- Right Knee Joint/LConn2
  Right Knee Joint/LConn3 -- Right Knee Sensor/LConn1
  Right Knee Joint/RConn1 -- Right Thigh Low/RConn1
  Right Knee Joint/RConn2 -- Right Knee IC/RConn1
  Right Thigh Sensor Sheet/LConn1 -- Right Thigh Low/LConn1
  Right Thigh High/RConn1 -- Right Thigh Sensor Sheet/RConn1
  HAT/RConn2 -- Right Heel Sensor9/LConn1
  Right Heel Sensor5/LConn1 -- HAT/LConn1
  Ground/LConn1 -- Machine Environment/RConn1
  Left Foot/LConn2 -- Left Ball Contact/LConn1
  Planar/LConn1 -- Ground/RConn1
  Planar/RConn1 -- Left Foot/LConn1
  HAT/RConn4 -- Right Hip Joint/RConn1
  HAT/RConn3 -- Right Heel Sensor8/LConn1
  Planar/LConn2 -- Left Ball IC/RConn1

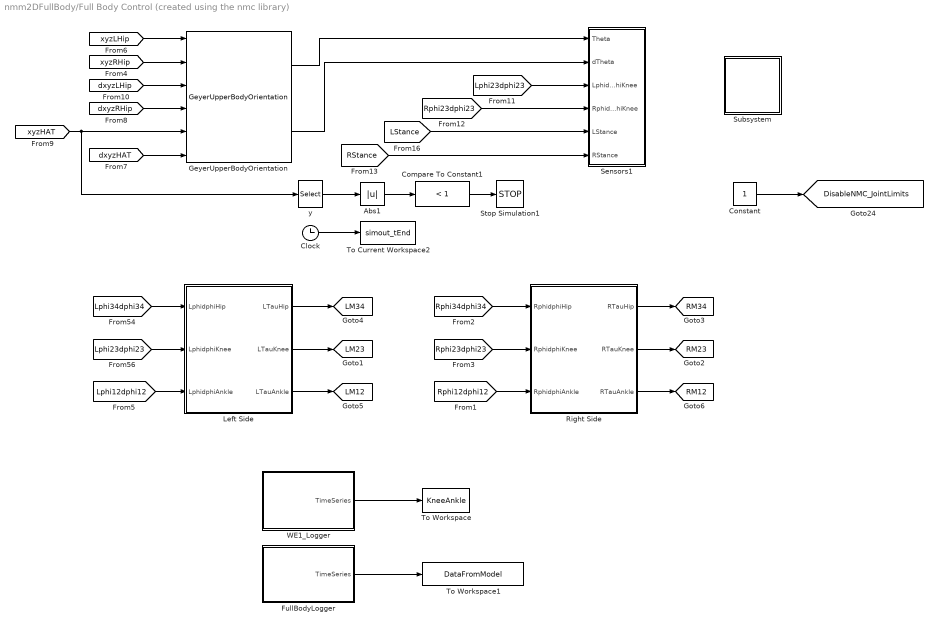
== system nmm2DFullBody/Full Body Control (created using the nmc library) ==
  " y" : Selector  InputPortWidth=3  IndexOptions=Index vector (dialog)  Indices=[2]  OutputSizes=1
  Abs1 : Abs
  Clock : Clock
  Compare To Constant1 : simulink/Logic and Bit Operations/Compare To Constant  relop=<  const=1  OutDataTypeStr=boolean
  Constant : Constant
  FullBodyLogger : Subsystem
  GeyerUpperBodyOrientation : nmc/NMC Sensors/GeyerUpperBodyOrientation
  Left Side : Subsystem  AncestorBlock=nmc/Full Body Control/Left Side
  Right Side : Subsystem  AncestorBlock=nmc/Full Body Control/Right Side
  Sensors1 : Subsystem  AncestorBlock=nmc/Sensors
  Stop Simulation1 : Stop
  Subsystem : Subsystem
  To Current Workspace2 : ToWorkspace  VariableName=simout_tEnd  SaveFormat=Structure  SampleTime=-1
      settings: MaxDataPoints=1
  To Workspace : ToWorkspace  VariableName=KneeAnkle  SaveFormat=Timeseries  SampleTime=0.001
  To Workspace1 : ToWorkspace  VariableName=DataFromModel  SaveFormat=Timeseries  SampleTime=0.001
  WE1_Logger : Subsystem
  tag scope: DisableNMC_JointLimits=global, LM12=global, LM23=global, LM34=global, RM12=global, RM23=global, RM34=global
  wires:
  [Lphi34dphi34] -> Left Side/1(LphidphiHip)
  [Lphi23dphi23] -> Left Side/2(LphidphiKnee)
  Left Side/1(LTauHip) -> [LM34]
  Left Side/2(LTauKnee) -> [LM23]
  Left Side/3(LTauAnkle) -> [LM12]
  [Lphi12dphi12] -> Left Side/3(LphidphiAnkle)
  [Rphi34dphi34] -> Right Side/1(RphidphiHip)
  [Rphi23dphi23] -> Right Side/2(RphidphiKnee)
  [Rphi12dphi12] -> Right Side/3(RphidphiAnkle)
  Right Side/1(RTauHip) -> [RM34]
  Right Side/2(RTauKnee) -> [RM23]
  Right Side/3(RTauAnkle) -> [RM12]
  [xyzLHip] -> GeyerUpperBodyOrientation/1
  [dxyzRHip] -> GeyerUpperBodyOrientation/4
  [dxyzHAT] -> GeyerUpperBodyOrientation/6
  [xyzRHip] -> GeyerUpperBodyOrientation/2
  [dxyzLHip] -> GeyerUpperBodyOrientation/3
  [xyzHAT] -> GeyerUpperBodyOrientation/5, " y"/1
  Clock/1 -> To Current Workspace2/1
  Abs1/1 -> Compare To Constant1/1
  Compare To Constant1/1 -> Stop Simulation1/1
  " y"/1 -> Abs1/1
  GeyerUpperBodyOrientation/1 -> Sensors1/1(Theta)
  GeyerUpperBodyOrientation/2 -> Sensors1/2(dTheta)
  [Lphi23dphi23] -> Sensors1/3(LphidphiKnee)
  [Rphi23dphi23] -> Sensors1/4(RphidphiKnee)
  [LStance] -> Sensors1/5(LStance)
  [RStance] -> Sensors1/6(RStance)
  Constant/1 -> [DisableNMC_JointLimits]
  WE1_Logger/1(TimeSeries) -> To Workspace/1
  FullBodyLogger/1(TimeSeries) -> To Workspace1/1

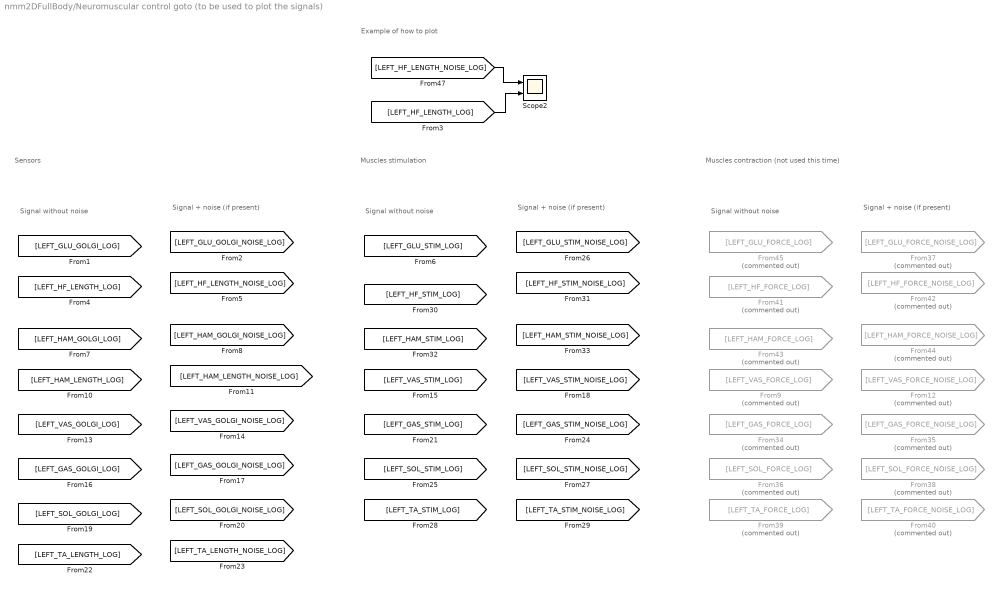
== system nmm2DFullBody/Neuromuscular control goto (to be used to plot the signals) ==
  note: Sensors
  note: Signal without noise
  note: Example of how to plot
  note: Signal + noise (if present)
  note: Muscles stimulation
  note: Signal without noise
  note: Signal + noise (if present)
  note: Muscles contraction (not used this time)
  note: Signal without noise
  note: Signal + noise (if present)
  From12 : From  Commented=on  GotoTag=LEFT_VAS_FORCE_NOISE_LOG  TagVisibility=global
  From34 : From  Commented=on  GotoTag=LEFT_GAS_FORCE_LOG  TagVisibility=global
  From35 : From  Commented=on  GotoTag=LEFT_GAS_FORCE_NOISE_LOG  TagVisibility=global
  From36 : From  Commented=on  GotoTag=LEFT_SOL_FORCE_LOG  TagVisibility=global
  From37 : From  Commented=on  GotoTag=LEFT_GLU_FORCE_NOISE_LOG  TagVisibility=global
  From38 : From  Commented=on  GotoTag=LEFT_SOL_FORCE_NOISE_LOG  TagVisibility=global
  From39 : From  Commented=on  GotoTag=LEFT_TA_FORCE_LOG  TagVisibility=global
  From40 : From  Commented=on  GotoTag=LEFT_TA_FORCE_NOISE_LOG  TagVisibility=global
  From41 : From  Commented=on  GotoTag=LEFT_HF_FORCE_LOG  TagVisibility=global
  From42 : From  Commented=on  GotoTag=LEFT_HF_FORCE_NOISE_LOG  TagVisibility=global
  From43 : From  Commented=on  GotoTag=LEFT_HAM_FORCE_LOG  TagVisibility=global
  From44 : From  Commented=on  GotoTag=LEFT_HAM_FORCE_NOISE_LOG  TagVisibility=global
  From45 : From  Commented=on  GotoTag=LEFT_GLU_FORCE_LOG  TagVisibility=global
  From9 : From  Commented=on  GotoTag=LEFT_VAS_FORCE_LOG  TagVisibility=global
  Scope2 : Scope  NumInputPorts=2
  wires:
  [LEFT_HF_LENGTH_LOG] -> Scope2/2
  [LEFT_HF_LENGTH_NOISE_LOG] -> Scope2/1
